simulink model "Brakes"  (R2014a)
settings: Solver=ode3  SolverMode=SingleTasking  StartTime=0.0  StopTime=inf  FixedStep=0.001  RelTol=1e-3
PreLoadFcn:
  | JR=0.8;%Mass Moment of Inertia Wheel [kg/m^2]
  | rR=0.3; %Wheel Radius [m]
  | cw=0.3; %Drag Coefficient[-]
  | A=2; %Frontal Area [m^2]
  | rho=1.2; %Air Density [kg/m^3]
  | m=1500; %Vehicle Mass [kg]
  | g=9.81; %Acceleration of Gravity [m/s^2]
  | c1=0.86;%Friction Coefficient Calculation [-]
  | c2=33.82; %Friction Coefficient Calculation [-]
  | c3=0.36;%Friction Coefficient Calculation [-]
undefined symbols (not defined in the file): v0
libraries: canoelib x9
settings Model: targetArch=x64  analysisModel=0  XcpMessageLength=-1  hasCAPLCallBlock=0  Creator=visjf  LastModifiedBy=vikafla
settings DataIOCC: SignalLoggingSaveFormat=ModelDataLogs
settings OptimizationCC: ExpressionDepthLimit=2147483647  InitFltsAndDblsToZero=on
settings DebuggingCC: SaveWithParameterizedLinksMsg=none  UnderspecifiedInitializationDetection=Classic  SignalResolutionControl=TryResolveAllWithWarning  SolverPrmCheckMsg=none  MultiTaskDSMMsg=warning  MultiTaskCondExecSysMsg=none  FcnCallInpInsideContextMsg=UseLocalSettings  StateNameClashWarn=warning
settings HardwareCC: TargetLongLongMode=on  TargetIntDivRoundTo=Zero  TargetEndianess=LittleEndian  TargetHWDeviceType=MATLAB Host  ProdEqTarget=off
settings RTWCC: SystemTargetFile=cn.tlc  TemplateMakefile=cn_msdll.tmf  ProcessScript=cn_make_rtw_hook  IncludeERTFirstTime=on
settings STFCustomTargetCC: TargetFcnLib=ansi_tfl_tmw.mat  ModelReferenceCompliant=off  ConcurrentExecutionCompliant=off  MatFileLogging=on  CPPClassGenCompliant=on  SystemTargetFile=cn.tlc
settings GRTTargetCC: TargetFcnLib=ansi_tfl_tmw.mat  ModelReferenceCompliant=off  ParMdlRefBuildCompliant=off  CompOptLevelCompliant=off  ConcurrentExecutionCompliant=off  CombineOutputUpdateFcns=off  GRTInterface=on  ExtModeMexFile=noextcomm  RTWCAPISignals=on  RTWCAPIParams=on

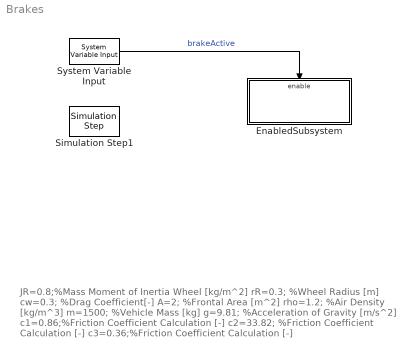
== system Brakes ==
  note: JR=0.8;%Mass Moment of Inertia Wheel [kg/m^2]
      | rR=0.3; %Wheel Radius [m]
      | cw=0.3; %Drag Coefficient[-]
      | A=2; %Frontal Area [m^2]
      | rho=1.2; %Air Density [kg/m^3]
      | m=1500; %Vehicle Mass [kg]
      | g=9.81; %Acceleration of Gravity [m/s^2]
      | c1=0.86;%Friction Coefficient Calculation [-]
      | c2=33.82; %Friction Coefficient Calculation [-]
      | c3=0.36;%Friction Coefficient Calculation [-]
  EnabledSubsystem : Subsystem  TreatAsAtomicUnit=on
  Simulation Step1 : canoelib/CANoe I//O/Simulation Step  mode=Offline
      settings: AttributesFormatString=%<mode>
  System Variable Input : canoelib/CANoe I//O/System Variable Input  nsName=Control  sysVarName=brakeActive  arrayIndex=-1  editSampleTime=0  rawValue=Default  dataType=Default  dataTypeDB=unknown  hasEncoding=off  dataTypeCANoe=Get from CANoe
      settings: AttributesFormatString=%<nsName>::%<sysVarName>
  wires:
  System Variable Input/1 -> EnabledSubsystem/Enable  "brakeActive"

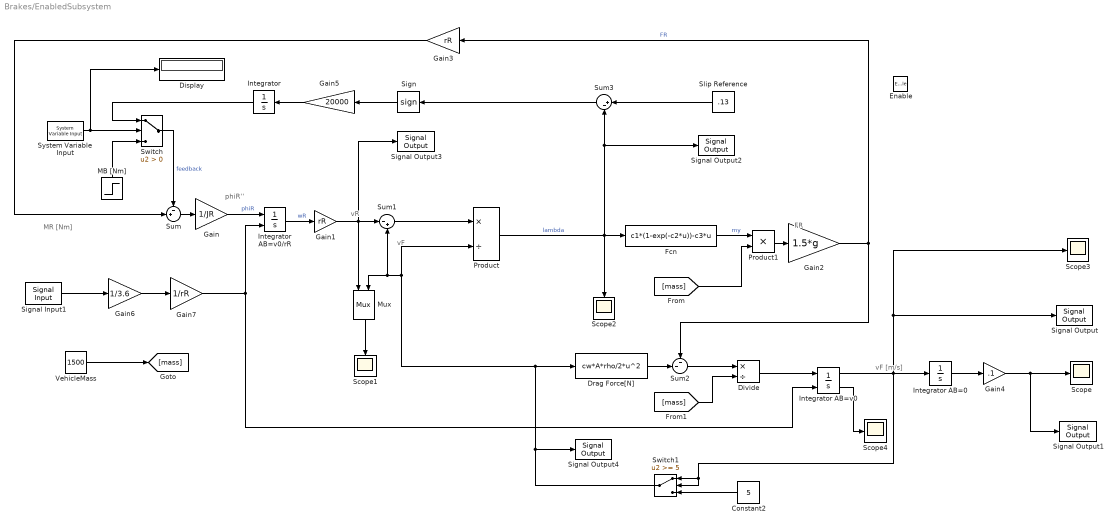
== system Brakes/EnabledSubsystem ==
  note: phiR''
  note: MR [Nm]
  note: vF
  note: vR
  note: vF [m/s]
  note: FR
  Enable : EnablePort  StatesWhenEnabling=reset
  Constant2 : Constant  Value=5
  Display : Display
  Divide : Product  Inputs=*/  RndMeth=Zero  InputSameDT=on  OutDataTypeStr=Inherit: Same as first input
  Drag Force[N] : Fcn  Expr=cw*A*rho/2*u^2
  Fcn : Fcn  Expr=c1*(1-exp(-c2*u))-c3*u
  Gain : Gain  Gain=1/JR  SaturateOnIntegerOverflow=on  OutDataTypeStr=Inherit: Same as input  ParamDataTypeStr=Inherit: Same as input
  Gain1 : Gain  Gain=rR  SaturateOnIntegerOverflow=on  OutDataTypeStr=Inherit: Same as input  ParamDataTypeStr=Inherit: Same as input
  Gain2 : Gain  Gain=1.5*g  SaturateOnIntegerOverflow=on  OutDataTypeStr=Inherit: Same as input  ParamDataTypeStr=Inherit: Same as input
  Gain3 : Gain  Gain=rR  SaturateOnIntegerOverflow=on  OutDataTypeStr=Inherit: Same as input  ParamDataTypeStr=Inherit: Same as input
  Gain4 : Gain  Gain=.1  OutDataTypeStr=Inherit: Same as input  ParamDataTypeStr=Inherit: Same as input
  Gain5 : Gain  Gain=20000  SaturateOnIntegerOverflow=on  OutDataTypeStr=Inherit: Same as input  ParamDataTypeStr=Inherit: Same as input
  Gain6 : Gain  Gain=1/3.6  OutDataTypeStr=Inherit: Same as input  ParamDataTypeStr=Inherit: Same as input
  Gain7 : Gain  Gain=1/rR  OutDataTypeStr=Inherit: Same as input  ParamDataTypeStr=Inherit: Same as input
  Integrator : Integrator  LimitOutput=on  LowerSaturationLimit=0
  Integrator AB=0 : Integrator  LimitOutput=on  LowerSaturationLimit=0
  Integrator AB=v0 : Integrator  InitialConditionSource=external  LimitOutput=on  LowerSaturationLimit=0  ShowSaturationPort=on
  Integrator AB=v0/rR : Integrator  InitialConditionSource=external  InitialCondition=v0/rR  LimitOutput=on  LowerSaturationLimit=0
  MB [Nm] : Step  Time=0  After=5355  SampleTime=0
  Mux : Mux  Inputs=2
      settings: DisplayOption=signals
  Product : Product  Inputs=*/  SaturateOnIntegerOverflow=on  RndMeth=Zero  InputSameDT=on  OutDataTypeStr=Inherit: Same as first input
  Product1 : Product  RndMeth=Zero  InputSameDT=on  OutDataTypeStr=Inherit: Same as first input
  Scope{,1..4} (5 alike) : Scope
      Scope settings: TimeRange=3  YMin=150  YMax=320  SaveName=x
      Scope1 settings: YMin=19  YMax=22.25  SaveName=v
      Scope2 settings: YMin=1  YMax=1  SaveName=lam
      Scope3 settings: TimeRange=3  YMin=17707.5  YMax=17716  SaveName=x1
      Scope4 settings: TimeRange=3  YMin=-1  YMax=1  SaveName=x2
  Sign : Signum
  Signal Input1 : canoelib/CANoe I//O/Signal Input  dbName=abs  nodeName=Chassis  msgName=MotorState  sigName=CarSpeed  editSampleTime=0  rawValue=Physical value  dataType=Default  dataTypeDB=unknown  hasEncoding=off
      settings: AttributesFormatString=%<sigName>
  Signal Output : canoelib/CANoe I//O/Signal Output  dbName=abs  nodeName=Chassis  msgName=MotorState  sigName=CarSpeed  rawValue=Physical value  dataType=Default  dataTypeDB=unknown  hasEncoding=off
      settings: AttributesFormatString=%<sigName>
  Signal Output1 : canoelib/CANoe I//O/Signal Output  dbName=""  nodeName=""  msgName=""  sigName=xF  rawValue=Physical value  dataType=Default  dataTypeDB=unknown  hasEncoding=off
      settings: AttributesFormatString=%<sigName>
  Signal Output2 : canoelib/CANoe I//O/Signal Output  dbName=""  nodeName=""  msgName=""  sigName=lambda  rawValue=Physical value  dataType=Default  dataTypeDB=unknown  hasEncoding=off
      settings: AttributesFormatString=%<sigName>
  Signal Output3 : canoelib/CANoe I//O/Signal Output  dbName=""  nodeName=""  msgName=""  sigName=vR  rawValue=Physical value  dataType=Default  dataTypeDB=unknown  hasEncoding=off
      settings: AttributesFormatString=%<sigName>
  Signal Output4 : canoelib/CANoe I//O/Signal Output  dbName=""  nodeName=""  msgName=""  sigName=vF  rawValue=Physical value  dataType=Default  dataTypeDB=unknown  hasEncoding=off
      settings: AttributesFormatString=%<sigName>
  Slip Reference : Constant  Value=.13
  Sum : Sum  Inputs=-+|  SaturateOnIntegerOverflow=on  InputSameDT=on  OutDataTypeStr=Inherit: Same as first input
  Sum1 : Sum  Inputs=|-+  SaturateOnIntegerOverflow=on  InputSameDT=on  OutDataTypeStr=Inherit: Same as first input
  Sum2 : Sum  Inputs=--|  SaturateOnIntegerOverflow=on  InputSameDT=on  OutDataTypeStr=Inherit: Same as first input
  Sum3 : Sum  Inputs=|+-  SaturateOnIntegerOverflow=on  InputSameDT=on  OutDataTypeStr=Inherit: Same as first input
  Switch : Switch  Criteria=u2 > Threshold  SaturateOnIntegerOverflow=on  InputSameDT=on
  Switch1 : Switch  Threshold=5  SaturateOnIntegerOverflow=on  InputSameDT=on
  System Variable Input : canoelib/CANoe I//O/System Variable Input  nsName=Control  sysVarName=activeABS  arrayIndex=-1  editSampleTime=0  rawValue=Default  dataType=Default  dataTypeDB=unknown  hasEncoding=off  dataTypeCANoe=Get from CANoe
      settings: AttributesFormatString=%<nsName>::%<sysVarName>
  VehicleMass : Constant  Value=1500
  wires:
  Integrator AB=v0/2 -> Scope4/1
  Gain7/1 -> Integrator AB=v0/rR/2, Integrator AB=v0/2
  Integrator AB=v0/rR/1 -> Gain1/1  "wR"
  Gain/1 -> Integrator AB=v0/rR/1  "phiR"
  Sum/1 -> Gain/1
  Switch1/1 -> Drag Force[N]/1, Product/2, Sum1/2, Mux/2, Signal Output4/1
  Constant2/1 -> Switch1/3
  Gain6/1 -> Gain7/1
  Sum3/1 -> Sign/1
  Sign/1 -> Gain5/1
  Gain5/1 -> Integrator/1
  Slip Reference/1 -> Sum3/1
  Mux/1 -> Scope1/1
  Gain1/1 -> Sum1/1, Mux/1, Signal Output3/1
  Product/1 -> Fcn/1, Sum3/2, Signal Output2/1, Scope2/1  "lambda"
  Integrator AB=0/1 -> Gain4/1
  Integrator AB=v0/1 -> Switch1/2, Switch1/1, Integrator AB=0/1, Signal Output/1, Scope3/1
  Gain2/1 -> Gain3/1, Sum2/1  "FR"
  Drag Force[N]/1 -> Sum2/2
  Sum1/1 -> Product/1
  Gain3/1 -> Sum/2
  Switch/1 -> Sum/1  "feedback"
  Integrator/1 -> Switch/1
  MB [Nm]/1 -> Switch/3
  System Variable Input/1 -> Switch/2, Display/1
  Signal Input1/1 -> Gain6/1
  VehicleMass/1 -> [mass]
  Fcn/1 -> Product1/1  "my"
  Product1/1 -> Gain2/1
  [mass] -> Product1/2
  Divide/1 -> Integrator AB=v0/1
  Sum2/1 -> Divide/1
  [mass] -> Divide/2
  Gain4/1 -> Scope/1, Signal Output1/1
